simulink model "t1q2"  (R2017b)
settings: Solver=VariableStepAuto  StartTime=0.0  StopTime=10.0  RelTol=1e-3
values from neighbouring files (symbols this model uses):
  k1 = 6.01    [t1.m]    (also in t1q5.m; t1q9.m)
  k2 = 0.8433    [t1.m]    (also in t1q5.m; t1q9.m)
  k3 = 0.1123    [t1.m]    (also in t1q5.m; t1q9.m)
settings Model: Creator=vinic  LastModifiedBy=vinic

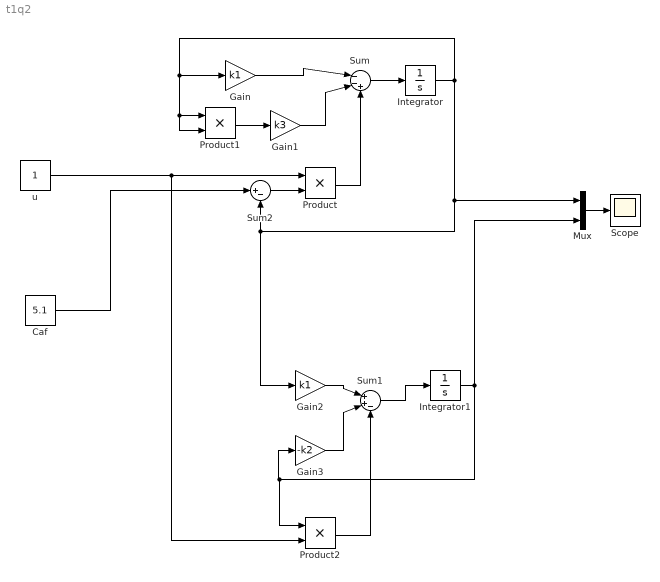
== system t1q2 ==
  Caf : Constant  Value=5.1
  Gain : Gain  Gain=k1
  Gain1 : Gain  Gain=k3
  Gain2 : Gain  Gain=k1
  Gain3 : Gain  Gain=-k2
  Integrator : Integrator
  Integrator1 : Integrator
  Mux : Mux  Inputs=2
  Product : Product
  Product1 : Product
  Product2 : Product
  Scope : Scope
  Sum : Sum  Inputs=|--+
  Sum1 : Sum  Inputs=|++-
  Sum2 : Sum  Inputs=|+-
  u : Constant
  wires:
  Caf/1 -> Sum2/1
  Integrator/1 -> Mux/1, Gain2/1, Sum2/2, Product1/1, Product1/2, Gain/1
  Sum2/1 -> Product/2
  u/1 -> Product2/2, Product/1
  Gain/1 -> Sum/1
  Product/1 -> Sum/3
  Sum/1 -> Integrator/1
  Integrator1/1 -> Mux/2, Product2/1, Gain3/1
  Gain2/1 -> Sum1/1
  Gain3/1 -> Sum1/2
  Product2/1 -> Sum1/3
  Sum1/1 -> Integrator1/1
  Mux/1 -> Scope/1
  Product1/1 -> Gain1/1
  Gain1/1 -> Sum/2
